simulink model "UserVehicle_RTW"  (Simulink 10.3)
settings: Solver=ode1  StartTime=0.0  StopTime=inf  FixedStep=0.001  RelTol=1e-3
PreLoadFcn:
  | vehicle = 'Car'; if ~length(which('cmcmd')), cmenv; end
  | UserVehicle_RTW_bus
  | UserVehicle_RTW_params
InitFcn:
  | vehicle = 'Car'; if ~length(which('cmcmd')), cmenv; end
  | UserVehicle_RTW_bus
undefined symbols (not defined in the file or in its folder): Car_Bdy1_mass, Car_Steering_i, Car_WhlBaseF, Car_WhlBaseR
libraries: CarMaker4SL x77
(part 1 of 3)
Description:
  | CarMaker Plug-in Model Target
settings Model: Creator=IPG  LastModifiedBy=IPG  MultithreadedSim=on
settings DataIOCC: LimitDataPoints=on
settings DebuggingCC: SFExecutionAtInitializationDiag=warning
settings HardwareCC: TargetHWDeviceType=32-bit Generic  ProdEqTarget=off
settings RTWCC: Description=CarMaker Plug-in Model Target  SystemTargetFile=CarMaker.tlc  TemplateMakefile=CarMaker_unix-win64.tmf
settings CodeAppCC: MaxIdLength=127
settings STFCustomTargetCC: ModelReferenceCompliant=off  CodeInterfacePackaging=Reusable function  CPPClassGenCompliant=on  GRTInterface=off  GenerateAllocFcn=on  SystemTargetFile=CarMaker.tlc
settings GRTTargetCC: ModelReferenceCompliant=off  ParMdlRefBuildCompliant=off  CompOptLevelCompliant=off  ConcurrentExecutionCompliant=off  MatFileLogging=off  CodeInterfacePackaging=Reusable function  GRTInterface=off  GenerateAllocFcn=on  UseToolchainInfoCompliant=off
settings CustomProperty: DataType=string
settings EnumStrPairs: String=Car

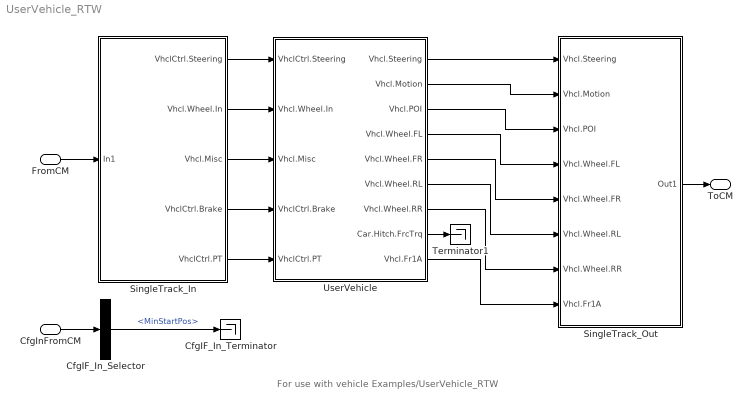
== system UserVehicle_RTW ==
  note: For use with vehicle Examples/UserVehicle_RTW
  FromCM : Inport  OutDataTypeStr=Bus: cmVehicle_CarIn
  CfgInFromCM : Inport  Port=2  OutDataTypeStr=Bus: cmVehicle_CarCfgIn
  CfgIF_In_Selector : BusSelector  OutputSignals=MinStartPos
  CfgIF_In_Terminator : Terminator
  SingleTrack_In : Subsystem
  SingleTrack_Out : Subsystem
  Terminator1 : Terminator
  UserVehicle : Subsystem
  ToCM : Outport  OutDataTypeStr=Bus: cmVehicle_CarOut  VectorParamsAs1DForOutWhenUnconnected=off
  wires:
  FromCM/1 -> SingleTrack_In/1(In1)
  SingleTrack_Out/1(Out1) -> ToCM/1
  CfgInFromCM/1 -> CfgIF_In_Selector/1
  CfgIF_In_Selector/1 -> CfgIF_In_Terminator/1  "<MinStartPos>"
  SingleTrack_In/1(VhclCtrl.Steering) -> UserVehicle/1(VhclCtrl.Steering)
  SingleTrack_In/2(Vhcl.Wheel.In) -> UserVehicle/2(Vhcl.Wheel.In)
  SingleTrack_In/3(Vhcl.Misc) -> UserVehicle/3(Vhcl.Misc)
  SingleTrack_In/4(VhclCtrl.Brake) -> UserVehicle/4(VhclCtrl.Brake)
  SingleTrack_In/5(VhclCtrl.PT) -> UserVehicle/5(VhclCtrl.PT)
  UserVehicle/1(Vhcl.Steering) -> SingleTrack_Out/1(Vhcl.Steering)
  UserVehicle/2(Vhcl.Motion) -> SingleTrack_Out/2(Vhcl.Motion)
  UserVehicle/3(Vhcl.POI) -> SingleTrack_Out/3(Vhcl.POI)
  UserVehicle/4(Vhcl.Wheel.FL) -> SingleTrack_Out/4(Vhcl.Wheel.FL)
  UserVehicle/5(Vhcl.Wheel.FR) -> SingleTrack_Out/5(Vhcl.Wheel.FR)
  UserVehicle/6(Vhcl.Wheel.RL) -> SingleTrack_Out/6(Vhcl.Wheel.RL)
  UserVehicle/7(Vhcl.Wheel.RR) -> SingleTrack_Out/7(Vhcl.Wheel.RR)
  UserVehicle/9(Vhcl.Fr1A) -> SingleTrack_Out/8(Vhcl.Fr1A)
  UserVehicle/8(Car.Hitch.FrcTrq) -> Terminator1/1

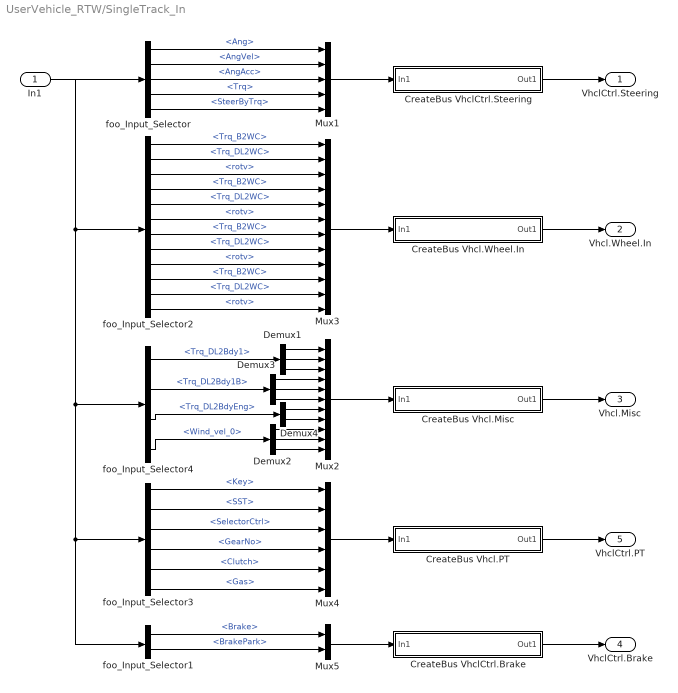
== system UserVehicle_RTW/SingleTrack_In ==
  In1 : Inport
  CreateBus Vhcl.Misc : Subsystem
  CreateBus Vhcl.PT : Subsystem
  CreateBus Vhcl.Wheel.In : Subsystem
  CreateBus VhclCtrl.Brake : Subsystem
  CreateBus VhclCtrl.Steering : Subsystem
  Demux1 : Demux  Outputs=3
      settings: DisplayOption=none
  Demux2 : Demux  Outputs=3
      settings: DisplayOption=none
  Demux3 : Demux  Outputs=3
      settings: DisplayOption=none
  Demux4 : Demux  Outputs=2
      settings: DisplayOption=none
  Mux1 : Mux  Inputs=5
  Mux2 : Mux  Inputs=11
  Mux3 : Mux  Inputs=12
  Mux4 : Mux  Inputs=6
  Mux5 : Mux  Inputs=2
  foo_Input_Selector : BusSelector  OutputSignals=VhclCtrl.Steering.Ang,VhclCtrl.Steering.AngVel,VhclCtrl.Steering.AngAcc,VhclCtrl.Steering.Trq,VhclCtrl.Steering.SteerByTrq
  foo_Input_Selector1 : BusSelector  OutputSignals=VhclCtrl.Brake,VhclCtrl.BrakePark
  foo_Input_Selector2 : BusSelector  OutputSignals=Vhcl.Wheel.FL.Trq_B2WC,Vhcl.Wheel.FL.Trq_DL2WC,Vhcl.Wheel.FL.rotv,Vhcl.Wheel.FR.Trq_B2WC,Vhcl.Wheel.FR.Trq_DL2WC,Vhcl.Wheel.FR.rotv,Vhcl.Wheel.RL.Trq_B2WC,Vhcl.Wheel.RL.Trq_DL2WC,Vhcl.Wheel.RL.rotv,Vhcl.Wheel.RR.Trq_B2WC,Vhcl.Wheel.RR.Trq_DL2WC,Vhcl.Wheel.RR.rotv
  foo_Input_Selector3 : BusSelector  OutputSignals=VhclCtrl.Key,VhclCtrl.SST,VhclCtrl.SelectorCtrl,VhclCtrl.GearNo,VhclCtrl.Clutch,VhclCtrl.Gas
  foo_Input_Selector4 : BusSelector  OutputSignals=Vhcl.Trq_DL2Bdy1,Vhcl.Trq_DL2Bdy1B,Vhcl.Trq_DL2BdyEng,Vhcl.Wind_vel_0
  VhclCtrl.Steering : Outport  VectorParamsAs1DForOutWhenUnconnected=off
  Vhcl.Wheel.In : Outport  Port=2  VectorParamsAs1DForOutWhenUnconnected=off
  Vhcl.Misc : Outport  Port=3  VectorParamsAs1DForOutWhenUnconnected=off
  VhclCtrl.Brake : Outport  Port=4  VectorParamsAs1DForOutWhenUnconnected=off
  VhclCtrl.PT : Outport  Port=5  VectorParamsAs1DForOutWhenUnconnected=off
  wires:
  foo_Input_Selector4/3 -> Demux4/1  "<Trq_DL2BdyEng>"
  Demux4/2 -> Mux2/8
  Demux4/1 -> Mux2/7
  foo_Input_Selector4/2 -> Demux3/1  "<Trq_DL2Bdy1B>"
  foo_Input_Selector4/1 -> Demux1/1  "<Trq_DL2Bdy1>"
  Demux3/3 -> Mux2/6
  Demux3/2 -> Mux2/5
  Demux3/1 -> Mux2/4
  Demux1/3 -> Mux2/3
  Demux1/2 -> Mux2/2
  Demux1/1 -> Mux2/1
  Demux2/3 -> Mux2/11
  Demux2/2 -> Mux2/10
  Demux2/1 -> Mux2/9
  foo_Input_Selector4/4 -> Demux2/1  "<Wind_vel_0>"
  foo_Input_Selector/5 -> Mux1/5  "<SteerByTrq>"
  In1/1 -> foo_Input_Selector4/1, foo_Input_Selector1/1, foo_Input_Selector3/1, foo_Input_Selector/1, foo_Input_Selector2/1
  foo_Input_Selector/1 -> Mux1/1  "<Ang>"
  foo_Input_Selector/2 -> Mux1/2  "<AngVel>"
  foo_Input_Selector/3 -> Mux1/3  "<AngAcc>"
  foo_Input_Selector/4 -> Mux1/4  "<Trq>"
  foo_Input_Selector2/1 -> Mux3/1  "<Trq_B2WC>"
  foo_Input_Selector2/2 -> Mux3/2  "<Trq_DL2WC>"
  foo_Input_Selector2/3 -> Mux3/3  "<rotv>"
  foo_Input_Selector2/4 -> Mux3/4  "<Trq_B2WC>"
  foo_Input_Selector2/5 -> Mux3/5  "<Trq_DL2WC>"
  foo_Input_Selector2/6 -> Mux3/6  "<rotv>"
  foo_Input_Selector2/7 -> Mux3/7  "<Trq_B2WC>"
  foo_Input_Selector2/8 -> Mux3/8  "<Trq_DL2WC>"
  foo_Input_Selector2/9 -> Mux3/9  "<rotv>"
  foo_Input_Selector2/10 -> Mux3/10  "<Trq_B2WC>"
  foo_Input_Selector2/11 -> Mux3/11  "<Trq_DL2WC>"
  foo_Input_Selector2/12 -> Mux3/12  "<rotv>"
  foo_Input_Selector1/1 -> Mux5/1  "<Brake>"
  Mux1/1 -> CreateBus VhclCtrl.Steering/1(In1)
  CreateBus VhclCtrl.Steering/1(Out1) -> VhclCtrl.Steering/1
  Mux3/1 -> CreateBus Vhcl.Wheel.In/1(In1)
  CreateBus Vhcl.Wheel.In/1(Out1) -> Vhcl.Wheel.In/1
  Mux2/1 -> CreateBus Vhcl.Misc/1(In1)
  CreateBus Vhcl.Misc/1(Out1) -> Vhcl.Misc/1
  Mux4/1 -> CreateBus Vhcl.PT/1(In1)
  CreateBus Vhcl.PT/1(Out1) -> VhclCtrl.PT/1
  Mux5/1 -> CreateBus VhclCtrl.Brake/1(In1)
  CreateBus VhclCtrl.Brake/1(Out1) -> VhclCtrl.Brake/1
  foo_Input_Selector1/2 -> Mux5/2  "<BrakePark>"
  foo_Input_Selector3/1 -> Mux4/1  "<Key>"
  foo_Input_Selector3/2 -> Mux4/2  "<SST>"
  foo_Input_Selector3/3 -> Mux4/3  "<SelectorCtrl>"
  foo_Input_Selector3/4 -> Mux4/4  "<GearNo>"
  foo_Input_Selector3/5 -> Mux4/5  "<Clutch>"
  foo_Input_Selector3/6 -> Mux4/6  "<Gas>"

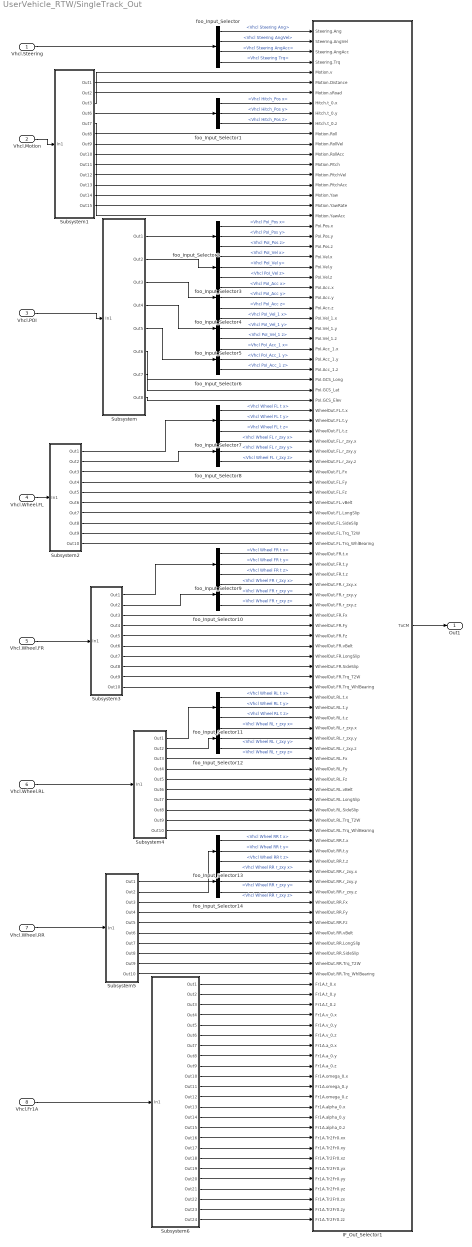
== system UserVehicle_RTW/SingleTrack_Out ==
  Vhcl.Steering : Inport
  Vhcl.Motion : Inport  Port=2
  Vhcl.POI : Inport  Port=3
  Vhcl.Wheel.FL : Inport  Port=4
  Vhcl.Wheel.FR : Inport  Port=5
  Vhcl.Wheel.RL : Inport  Port=6
  Vhcl.Wheel.RR : Inport  Port=7
  Vhcl.Fr1A : Inport  Port=8
  IF_Out_Selector1 : Subsystem  mask(Signal Selection){}
      mask help: Signal Selection Block
      settings: OpenFcn=cmSignalSelect('SignalSelection_CB',gcb)
  Subsystem : Subsystem
  Subsystem1 : Subsystem
  Subsystem2 : Subsystem
  Subsystem3 : Subsystem
  Subsystem4 : Subsystem
  Subsystem5 : Subsystem
  Subsystem6 : Subsystem
  foo_Input_Selector : BusSelector  OutputSignals=Vhcl Steering Ang,Vhcl Steering AngVel,Vhcl Steering AngAcc,Vhcl Steering Trq
  foo_Input_Selector1 : BusSelector  OutputSignals=Vhcl Hitch_Pos x,Vhcl Hitch_Pos y,Vhcl Hitch_Pos z
  foo_Input_Selector10 : BusSelector  OutputSignals=Vhcl Wheel FR r_zxy x,Vhcl Wheel FR r_zxy y,Vhcl Wheel FR r_zxy z
  foo_Input_Selector11 : BusSelector  OutputSignals=Vhcl Wheel RL t x,Vhcl Wheel RL t y,Vhcl Wheel RL t z
  foo_Input_Selector12 : BusSelector  OutputSignals=Vhcl Wheel RL r_zxy x,Vhcl Wheel RL r_zxy y,Vhcl Wheel RL r_zxy z
  foo_Input_Selector13 : BusSelector  OutputSignals=Vhcl Wheel RR t x,Vhcl Wheel RR t y,Vhcl Wheel RR t z
  foo_Input_Selector14 : BusSelector  OutputSignals=Vhcl Wheel RR r_zxy x,Vhcl Wheel RR r_zxy y,Vhcl Wheel RR r_zxy z
  foo_Input_Selector2 : BusSelector  OutputSignals=Vhcl PoI_Pos x,Vhcl PoI_Pos y,Vhcl PoI_Pos z
  foo_Input_Selector3 : BusSelector  OutputSignals=Vhcl PoI_Vel x,Vhcl PoI_Vel y,Vhcl PoI_Vel z
  foo_Input_Selector4 : BusSelector  OutputSignals=Vhcl PoI_Acc x,Vhcl PoI_Acc y,Vhcl PoI_Acc z
  foo_Input_Selector5 : BusSelector  OutputSignals=Vhcl PoI_Vel_1 x,Vhcl PoI_Vel_1 y,Vhcl PoI_Vel_1 z
  foo_Input_Selector6 : BusSelector  OutputSignals=Vhcl PoI_Acc_1 x,Vhcl PoI_Acc_1 y,Vhcl PoI_Acc_1 z
  foo_Input_Selector7 : BusSelector  OutputSignals=Vhcl Wheel FL t x,Vhcl Wheel FL t y,Vhcl Wheel FL t z
  foo_Input_Selector8 : BusSelector  OutputSignals=Vhcl Wheel FL r_zxy x,Vhcl Wheel FL r_zxy y,Vhcl Wheel FL r_zxy z
  foo_Input_Selector9 : BusSelector  OutputSignals=Vhcl Wheel FR t x,Vhcl Wheel FR t y,Vhcl Wheel FR t z
  Out1 : Outport  VectorParamsAs1DForOutWhenUnconnected=off
  wires:
  Subsystem5/2(Out2) -> foo_Input_Selector14/1
  Subsystem5/1(Out1) -> foo_Input_Selector13/1
  Subsystem4/2(Out2) -> foo_Input_Selector12/1
  Subsystem4/1(Out1) -> foo_Input_Selector11/1
  Subsystem3/2(Out2) -> foo_Input_Selector10/1
  Subsystem3/1(Out1) -> foo_Input_Selector9/1
  Subsystem2/2(Out2) -> foo_Input_Selector8/1
  Subsystem2/1(Out1) -> foo_Input_Selector7/1
  Subsystem/5(Out5) -> foo_Input_Selector6/1
  Subsystem/4(Out4) -> foo_Input_Selector5/1
  Subsystem/3(Out3) -> foo_Input_Selector4/1
  Subsystem/2(Out2) -> foo_Input_Selector3/1
  Subsystem/1(Out1) -> foo_Input_Selector2/1
  Vhcl.Steering/1 -> foo_Input_Selector/1
  Vhcl.Motion/1 -> Subsystem1/1(In1)
  Vhcl.POI/1 -> Subsystem/1(In1)
  Vhcl.Wheel.FL/1 -> Subsystem2/1(In1)
  Vhcl.Wheel.FR/1 -> Subsystem3/1(In1)
  Vhcl.Wheel.RL/1 -> Subsystem4/1(In1)
  Vhcl.Wheel.RR/1 -> Subsystem5/1(In1)
  Vhcl.Fr1A/1 -> Subsystem6/1(In1)
  Subsystem1/4(Out6) -> foo_Input_Selector1/1
  foo_Input_Selector/1 -> IF_Out_Selector1/1(Steering.Ang)  "<Vhcl Steering Ang>"
  foo_Input_Selector/2 -> IF_Out_Selector1/2(Steering.AngVel)  "<Vhcl Steering AngVel>"
  foo_Input_Selector/3 -> IF_Out_Selector1/3(Steering.AngAcc)  "<Vhcl Steering AngAcc>"
  foo_Input_Selector/4 -> IF_Out_Selector1/4(Steering.Trq)  "<Vhcl Steering Trq>"
  Subsystem1/1(Out1) -> IF_Out_Selector1/5(Motion.v)
  Subsystem1/2(Out2) -> IF_Out_Selector1/6(Motion.Distance)
  Subsystem1/3(Out3) -> IF_Out_Selector1/7(Motion.sRoad)
  foo_Input_Selector1/1 -> IF_Out_Selector1/8(Hitch.t_0.x)  "<Vhcl Hitch_Pos x>"
  foo_Input_Selector1/2 -> IF_Out_Selector1/9(Hitch.t_0.y)  "<Vhcl Hitch_Pos y>"
  foo_Input_Selector1/3 -> IF_Out_Selector1/10(Hitch.t_0.z)  "<Vhcl Hitch_Pos z>"
  Subsystem1/5(Out7) -> IF_Out_Selector1/11(Motion.Roll)
  Subsystem1/6(Out8) -> IF_Out_Selector1/12(Motion.RollVel)
  Subsystem1/7(Out9) -> IF_Out_Selector1/13(Motion.RollAcc)
  Subsystem1/8(Out10) -> IF_Out_Selector1/14(Motion.Pitch)
  Subsystem1/9(Out11) -> IF_Out_Selector1/15(Motion.PitchVel)
  Subsystem1/10(Out12) -> IF_Out_Selector1/16(Motion.PitchAcc)
  Subsystem1/11(Out13) -> IF_Out_Selector1/17(Motion.Yaw)
  Subsystem1/12(Out14) -> IF_Out_Selector1/18(Motion.YawRate)
  Subsystem1/13(Out15) -> IF_Out_Selector1/19(Motion.YawAcc)
  foo_Input_Selector2/1 -> IF_Out_Selector1/20(PoI.Pos.x)  "<Vhcl PoI_Pos x>"
  foo_Input_Selector2/2 -> IF_Out_Selector1/21(PoI.Pos.y)  "<Vhcl PoI_Pos y>"
  foo_Input_Selector2/3 -> IF_Out_Selector1/22(PoI.Pos.z)  "<Vhcl PoI_Pos z>"
  foo_Input_Selector3/1 -> IF_Out_Selector1/23(PoI.Vel.x)  "<Vhcl PoI_Vel x>"
  foo_Input_Selector3/2 -> IF_Out_Selector1/24(PoI.Vel.y)  "<Vhcl PoI_Vel y>"
  foo_Input_Selector3/3 -> IF_Out_Selector1/25(PoI.Vel.z)  "<Vhcl PoI_Vel z>"
  foo_Input_Selector4/1 -> IF_Out_Selector1/26(PoI.Acc.x)  "<Vhcl PoI_Acc x>"
  foo_Input_Selector4/2 -> IF_Out_Selector1/27(PoI.Acc.y)  "<Vhcl PoI_Acc y>"
  foo_Input_Selector4/3 -> IF_Out_Selector1/28(PoI.Acc.z)  "<Vhcl PoI_Acc z>"
  foo_Input_Selector5/1 -> IF_Out_Selector1/29(PoI.Vel_1.x)  "<Vhcl PoI_Vel_1 x>"
  foo_Input_Selector5/2 -> IF_Out_Selector1/30(PoI.Vel_1.y)  "<Vhcl PoI_Vel_1 y>"
  foo_Input_Selector5/3 -> IF_Out_Selector1/31(PoI.Vel_1.z)  "<Vhcl PoI_Vel_1 z>"
  foo_Input_Selector6/1 -> IF_Out_Selector1/32(PoI.Acc_1.x)  "<Vhcl PoI_Acc_1 x>"
  foo_Input_Selector6/2 -> IF_Out_Selector1/33(PoI.Acc_1.y)  "<Vhcl PoI_Acc_1 y>"
  foo_Input_Selector6/3 -> IF_Out_Selector1/34(PoI.Acc_1.z)  "<Vhcl PoI_Acc_1 z>"
  Subsystem/6(Out6) -> IF_Out_Selector1/35(PoI.GCS_Long)
  Subsystem/7(Out7) -> IF_Out_Selector1/36(PoI.GCS_Lat)
  Subsystem/8(Out8) -> IF_Out_Selector1/37(PoI.GCS_Elev)
  foo_Input_Selector7/1 -> IF_Out_Selector1/38(WheelOut.FL.t.x)  "<Vhcl Wheel FL t x>"
  foo_Input_Selector7/2 -> IF_Out_Selector1/39(WheelOut.FL.t.y)  "<Vhcl Wheel FL t y>"
  foo_Input_Selector7/3 -> IF_Out_Selector1/40(WheelOut.FL.t.z)  "<Vhcl Wheel FL t z>"
  foo_Input_Selector8/1 -> IF_Out_Selector1/41(WheelOut.FL.r_zxy.x)  "<Vhcl Wheel FL r_zxy x>"
  foo_Input_Selector8/2 -> IF_Out_Selector1/42(WheelOut.FL.r_zxy.y)  "<Vhcl Wheel FL r_zxy y>"
  foo_Input_Selector8/3 -> IF_Out_Selector1/43(WheelOut.FL.r_zxy.z)  "<Vhcl Wheel FL r_zxy z>"
  Subsystem2/3(Out3) -> IF_Out_Selector1/44(WheelOut.FL.Fx)
  Subsystem2/4(Out4) -> IF_Out_Selector1/45(WheelOut.FL.Fy)
  Subsystem2/5(Out5) -> IF_Out_Selector1/46(WheelOut.FL.Fz)
  Subsystem2/6(Out6) -> IF_Out_Selector1/47(WheelOut.FL.vBelt)
  Subsystem2/7(Out7) -> IF_Out_Selector1/48(WheelOut.FL.LongSlip)
  Subsystem2/8(Out8) -> IF_Out_Selector1/49(WheelOut.FL.SideSlip)
  Subsystem2/9(Out9) -> IF_Out_Selector1/50(WheelOut.FL.Trq_T2W)
  Subsystem2/10(Out10) -> IF_Out_Selector1/51(WheelOut.FL.Trq_WhlBearing)
  foo_Input_Selector9/1 -> IF_Out_Selector1/52(WheelOut.FR.t.x)  "<Vhcl Wheel FR t x>"
  foo_Input_Selector9/2 -> IF_Out_Selector1/53(WheelOut.FR.t.y)  "<Vhcl Wheel FR t y>"
  foo_Input_Selector9/3 -> IF_Out_Selector1/54(WheelOut.FR.t.z)  "<Vhcl Wheel FR t z>"
  foo_Input_Selector10/1 -> IF_Out_Selector1/55(WheelOut.FR.r_zxy.x)  "<Vhcl Wheel FR r_zxy x>"
  foo_Input_Selector10/2 -> IF_Out_Selector1/56(WheelOut.FR.r_zxy.y)  "<Vhcl Wheel FR r_zxy y>"
  foo_Input_Selector10/3 -> IF_Out_Selector1/57(WheelOut.FR.r_zxy.z)  "<Vhcl Wheel FR r_zxy z>"
  Subsystem3/3(Out3) -> IF_Out_Selector1/58(WheelOut.FR.Fx)
  Subsystem3/4(Out4) -> IF_Out_Selector1/59(WheelOut.FR.Fy)
  Subsystem3/5(Out5) -> IF_Out_Selector1/60(WheelOut.FR.Fz)
  Subsystem3/6(Out6) -> IF_Out_Selector1/61(WheelOut.FR.vBelt)
  Subsystem3/7(Out7) -> IF_Out_Selector1/62(WheelOut.FR.LongSlip)
  Subsystem3/8(Out8) -> IF_Out_Selector1/63(WheelOut.FR.SideSlip)
  Subsystem3/9(Out9) -> IF_Out_Selector1/64(WheelOut.FR.Trq_T2W)
  Subsystem3/10(Out10) -> IF_Out_Selector1/65(WheelOut.FR.Trq_WhlBearing)
  foo_Input_Selector11/1 -> IF_Out_Selector1/66(WheelOut.RL.t.x)  "<Vhcl Wheel RL t x>"
  foo_Input_Selector11/2 -> IF_Out_Selector1/67(WheelOut.RL.t.y)  "<Vhcl Wheel RL t y>"
  foo_Input_Selector11/3 -> IF_Out_Selector1/68(WheelOut.RL.t.z)  "<Vhcl Wheel RL t z>"
  foo_Input_Selector12/1 -> IF_Out_Selector1/69(WheelOut.RL.r_zxy.x)  "<Vhcl Wheel RL r_zxy x>"
  foo_Input_Selector12/2 -> IF_Out_Selector1/70(WheelOut.RL.r_zxy.y)  "<Vhcl Wheel RL r_zxy y>"
  foo_Input_Selector12/3 -> IF_Out_Selector1/71(WheelOut.RL.r_zxy.z)  "<Vhcl Wheel RL r_zxy z>"
  Subsystem4/3(Out3) -> IF_Out_Selector1/72(WheelOut.RL.Fx)
  Subsystem4/4(Out4) -> IF_Out_Selector1/73(WheelOut.RL.Fy)
  Subsystem4/5(Out5) -> IF_Out_Selector1/74(WheelOut.RL.Fz)
  Subsystem4/6(Out6) -> IF_Out_Selector1/75(WheelOut.RL.vBelt)
  Subsystem4/7(Out7) -> IF_Out_Selector1/76(WheelOut.RL.LongSlip)
  Subsystem4/8(Out8) -> IF_Out_Selector1/77(WheelOut.RL.SideSlip)
  Subsystem4/9(Out9) -> IF_Out_Selector1/78(WheelOut.RL.Trq_T2W)
  Subsystem4/10(Out10) -> IF_Out_Selector1/79(WheelOut.RL.Trq_WhlBearing)
  foo_Input_Selector13/1 -> IF_Out_Selector1/80(WheelOut.RR.t.x)  "<Vhcl Wheel RR t x>"
  foo_Input_Selector13/2 -> IF_Out_Selector1/81(WheelOut.RR.t.y)  "<Vhcl Wheel RR t y>"
  foo_Input_Selector13/3 -> IF_Out_Selector1/82(WheelOut.RR.t.z)  "<Vhcl Wheel RR t z>"
  foo_Input_Selector14/1 -> IF_Out_Selector1/83(WheelOut.RR.r_zxy.x)  "<Vhcl Wheel RR r_zxy x>"
  foo_Input_Selector14/2 -> IF_Out_Selector1/84(WheelOut.RR.r_zxy.y)  "<Vhcl Wheel RR r_zxy y>"
  foo_Input_Selector14/3 -> IF_Out_Selector1/85(WheelOut.RR.r_zxy.z)  "<Vhcl Wheel RR r_zxy z>"
  Subsystem5/3(Out3) -> IF_Out_Selector1/86(WheelOut.RR.Fx)
  Subsystem5/4(Out4) -> IF_Out_Selector1/87(WheelOut.RR.Fy)
  Subsystem5/5(Out5) -> IF_Out_Selector1/88(WheelOut.RR.Fz)
  Subsystem5/6(Out6) -> IF_Out_Selector1/89(WheelOut.RR.vBelt)
  Subsystem5/7(Out7) -> IF_Out_Selector1/90(WheelOut.RR.LongSlip)
  Subsystem5/8(Out8) -> IF_Out_Selector1/91(WheelOut.RR.SideSlip)
  Subsystem5/9(Out9) -> IF_Out_Selector1/92(WheelOut.RR.Trq_T2W)
  Subsystem5/10(Out10) -> IF_Out_Selector1/93(WheelOut.RR.Trq_WhlBearing)
  Subsystem6/1(Out1) -> IF_Out_Selector1/94(Fr1A.t_0.x)
  Subsystem6/2(Out2) -> IF_Out_Selector1/95(Fr1A.t_0.y)
  Subsystem6/3(Out3) -> IF_Out_Selector1/96(Fr1A.t_0.z)
  Subsystem6/4(Out4) -> IF_Out_Selector1/97(Fr1A.v_0.x)
  Subsystem6/5(Out5) -> IF_Out_Selector1/98(Fr1A.v_0.y)
  Subsystem6/6(Out6) -> IF_Out_Selector1/99(Fr1A.v_0.z)
  Subsystem6/7(Out7) -> IF_Out_Selector1/100(Fr1A.a_0.x)
  Subsystem6/8(Out8) -> IF_Out_Selector1/101(Fr1A.a_0.y)
  Subsystem6/9(Out9) -> IF_Out_Selector1/102(Fr1A.a_0.z)
  Subsystem6/10(Out10) -> IF_Out_Selector1/103(Fr1A.omega_0.x)
  Subsystem6/11(Out11) -> IF_Out_Selector1/104(Fr1A.omega_0.y)
  Subsystem6/12(Out12) -> IF_Out_Selector1/105(Fr1A.omega_0.z)
  Subsystem6/13(Out13) -> IF_Out_Selector1/106(Fr1A.alpha_0.x)
  Subsystem6/14(Out14) -> IF_Out_Selector1/107(Fr1A.alpha_0.y)
  Subsystem6/15(Out15) -> IF_Out_Selector1/108(Fr1A.alpha_0.z)
  Subsystem6/16(Out16) -> IF_Out_Selector1/109(Fr1A.Tr2Fr0.xx)
  Subsystem6/17(Out17) -> IF_Out_Selector1/110(Fr1A.Tr2Fr0.xy)
  Subsystem6/18(Out18) -> IF_Out_Selector1/111(Fr1A.Tr2Fr0.xz)
  Subsystem6/19(Out19) -> IF_Out_Selector1/112(Fr1A.Tr2Fr0.yx)
  Subsystem6/20(Out20) -> IF_Out_Selector1/113(Fr1A.Tr2Fr0.yy)
  Subsystem6/21(Out21) -> IF_Out_Selector1/114(Fr1A.Tr2Fr0.yz)
  Subsystem6/22(Out22) -> IF_Out_Selector1/115(Fr1A.Tr2Fr0.zx)
  Subsystem6/23(Out23) -> IF_Out_Selector1/116(Fr1A.Tr2Fr0.zy)
  Subsystem6/24(Out24) -> IF_Out_Selector1/117(Fr1A.Tr2Fr0.zz)
  IF_Out_Selector1/1(ToCM) -> Out1/1

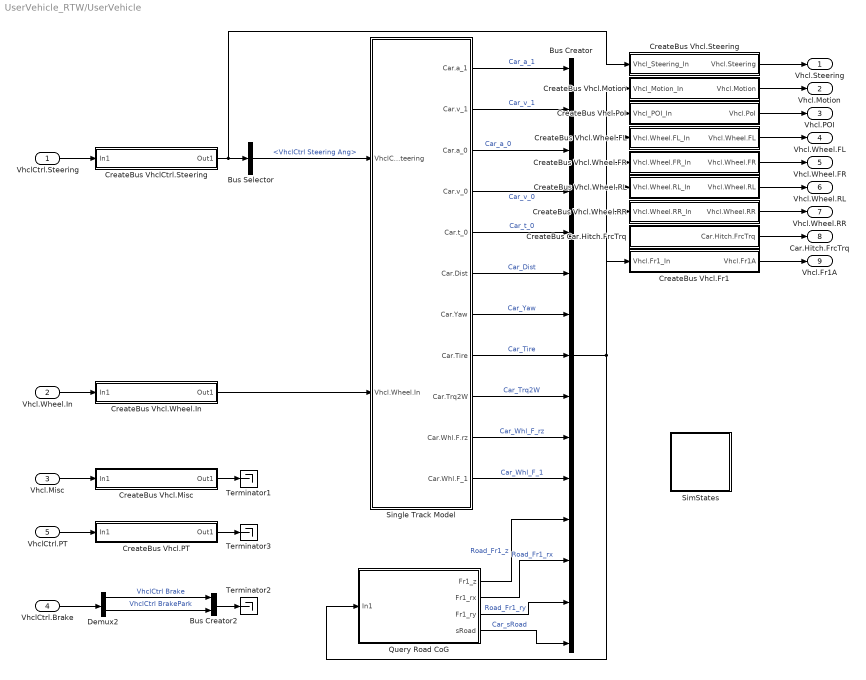
== system UserVehicle_RTW/UserVehicle ==
  VhclCtrl.Steering : Inport  OutDataTypeStr=double  BusOutputAsStruct=on
  Vhcl.Wheel.In : Inport  Port=2
  Vhcl.Misc : Inport  Port=3
  VhclCtrl.Brake : Inport  Port=4
  VhclCtrl.PT : Inport  Port=5
  Bus Creator : BusCreator  Inputs=15
  Bus Creator2 : BusCreator  Inputs=2
  Bus Selector : BusSelector  OutputSignals=VhclCtrl Steering Ang
  CreateBus Car.Hitch.FrcTrq : Subsystem
  CreateBus Vhcl.Fr1 : Subsystem
  CreateBus Vhcl.Misc : Subsystem
  CreateBus Vhcl.Motion : Subsystem
  CreateBus Vhcl.PT : Subsystem
  CreateBus Vhcl.PoI : Subsystem
  CreateBus Vhcl.Steering : Subsystem
  CreateBus Vhcl.Wheel.FL : Subsystem
  CreateBus Vhcl.Wheel.FR : Subsystem
  CreateBus Vhcl.Wheel.In : Subsystem
  CreateBus Vhcl.Wheel.RL : Subsystem
  CreateBus Vhcl.Wheel.RR : Subsystem
  CreateBus VhclCtrl.Steering : Subsystem
  Demux2 : Demux  Outputs=2
      settings: DisplayOption=none
  Query Road CoG : Subsystem
  SimStates : Subsystem
  Single Track Model : Subsystem
  Terminator1 : Terminator
  Terminator2 : Terminator
  Terminator3 : Terminator
  Vhcl.Steering : Outport  VectorParamsAs1DForOutWhenUnconnected=off
  Vhcl.Motion : Outport  Port=2  VectorParamsAs1DForOutWhenUnconnected=off
  Vhcl.POI : Outport  Port=3  VectorParamsAs1DForOutWhenUnconnected=off
  Vhcl.Wheel.FL : Outport  Port=4  VectorParamsAs1DForOutWhenUnconnected=off
  Vhcl.Wheel.FR : Outport  Port=5  VectorParamsAs1DForOutWhenUnconnected=off
  Vhcl.Wheel.RL : Outport  Port=6  VectorParamsAs1DForOutWhenUnconnected=off
  Vhcl.Wheel.RR : Outport  Port=7  VectorParamsAs1DForOutWhenUnconnected=off
  Car.Hitch.FrcTrq : Outport  Port=8  VectorParamsAs1DForOutWhenUnconnected=off
  Vhcl.Fr1A : Outport  Port=9  VectorParamsAs1DForOutWhenUnconnected=off
  wires:
  CreateBus Vhcl.Wheel.In/1(Out1) -> Single Track Model/2(Vhcl.Wheel.In)
  Single Track Model/11(Car.Whl.F_1) -> Bus Creator/11  "Car_Whl_F_1"
  Query Road CoG/4(sRoad) -> Bus Creator/15  "Car_sRoad"
  Query Road CoG/3(Fr1_ry) -> Bus Creator/14  "Road_Fr1_ry"
  Query Road CoG/2(Fr1_rx) -> Bus Creator/13  "Road_Fr1_rx"
  Query Road CoG/1(Fr1_z) -> Bus Creator/12  "Road_Fr1_z"
  Single Track Model/10(Car.Whl.F.rz) -> Bus Creator/10  "Car_Whl_F_rz"
  Bus Selector/1 -> Single Track Model/1(VhclCtrl.Steering)  "<VhclCtrl Steering Ang>"
  Single Track Model/1(Car.a_1) -> Bus Creator/1  "Car_a_1"
  Single Track Model/2(Car.v_1) -> Bus Creator/2  "Car_v_1"
  Single Track Model/3(Car.a_0) -> Bus Creator/3  "Car_a_0"
  Single Track Model/4(Car.v_0) -> Bus Creator/4  "Car_v_0"
  Single Track Model/5(Car.t_0) -> Bus Creator/5  "Car_t_0"
  Single Track Model/6(Car.Dist) -> Bus Creator/6  "Car_Dist"
  Single Track Model/7(Car.Yaw) -> Bus Creator/7  "Car_Yaw"
  Single Track Model/8(Car.Tire) -> Bus Creator/8  "Car_Tire"
  Single Track Model/9(Car.Trq2W) -> Bus Creator/9  "Car_Trq2W"
  Bus Creator/1 -> CreateBus Vhcl.Motion/1(Vhcl_Motion_In), CreateBus Vhcl.Wheel.RR/1(Vhcl.Wheel.RR_In), CreateBus Vhcl.Wheel.RL/1(Vhcl.Wheel.RL_In), CreateBus Vhcl.Wheel.FR/1(Vhcl.Wheel.FR_In), CreateBus Vhcl.Wheel.FL/1(Vhcl.Wheel.FL_In), CreateBus Vhcl.Fr1/1(Vhcl.Fr1_In), Query Road CoG/1(In1), CreateBus Vhcl.PoI/1(Vhcl_POI_In)
  CreateBus Vhcl.PT/1(Out1) -> Terminator3/1
  Bus Creator2/1 -> Terminator2/1
  CreateBus Vhcl.Misc/1(Out1) -> Terminator1/1
  VhclCtrl.Brake/1 -> Demux2/1
  Demux2/2 -> Bus Creator2/2  "VhclCtrl BrakePark"
  Demux2/1 -> Bus Creator2/1  "VhclCtrl Brake"
  CreateBus VhclCtrl.Steering/1(Out1) -> CreateBus Vhcl.Steering/1(Vhcl_Steering_In), Bus Selector/1
  VhclCtrl.Steering/1 -> CreateBus VhclCtrl.Steering/1(In1)
  Vhcl.Wheel.In/1 -> CreateBus Vhcl.Wheel.In/1(In1)
  Vhcl.Misc/1 -> CreateBus Vhcl.Misc/1(In1)
  CreateBus Vhcl.Steering/1(Vhcl.Steering) -> Vhcl.Steering/1
  CreateBus Vhcl.Wheel.RR/1(Vhcl.Wheel.RR) -> Vhcl.Wheel.RR/1
  CreateBus Car.Hitch.FrcTrq/1(Car.Hitch.FrcTrq) -> Car.Hitch.FrcTrq/1
  VhclCtrl.PT/1 -> CreateBus Vhcl.PT/1(In1)
  CreateBus Vhcl.Wheel.RL/1(Vhcl.Wheel.RL) -> Vhcl.Wheel.RL/1
  CreateBus Vhcl.Wheel.FR/1(Vhcl.Wheel.FR) -> Vhcl.Wheel.FR/1
  CreateBus Vhcl.Wheel.FL/1(Vhcl.Wheel.FL) -> Vhcl.Wheel.FL/1
  CreateBus Vhcl.PoI/1(Vhcl.PoI) -> Vhcl.POI/1
  CreateBus Vhcl.Motion/1(Vhcl.Motion) -> Vhcl.Motion/1
  CreateBus Vhcl.Fr1/1(Vhcl.Fr1A) -> Vhcl.Fr1A/1

== system UserVehicle_RTW/SingleTrack_In/CreateBus Vhcl.Misc ==
  In1 : Inport
  Bus Creator5 : BusCreator  Inputs=11
  Demux5 : Demux  Outputs=11
      settings: DisplayOption=none
  Out1 : Outport  VectorParamsAs1DForOutWhenUnconnected=off
  wires:
  Demux5/1 -> Bus Creator5/1  "Vhcl Trq_DL2Bdy1 x"
  Demux5/2 -> Bus Creator5/2  "Vhcl Trq_DL2Bdy1 y"
  Bus Creator5/1 -> Out1/1
  In1/1 -> Demux5/1
  Demux5/3 -> Bus Creator5/3  "Vhcl Trq_DL2Bdy1 z"
  Demux5/4 -> Bus Creator5/4  "Vhcl TrqDL2Bdy1B x"
  Demux5/5 -> Bus Creator5/5  "Vhcl TrqDL2Bdy1B y"
  Demux5/6 -> Bus Creator5/6  "Vhcl TrqDL2Bdy1B z"
  Demux5/7 -> Bus Creator5/7  "Vhcl DL2BdyEng x"
  Demux5/8 -> Bus Creator5/8  "Vhcl DL2BdyEng y"
  Demux5/9 -> Bus Creator5/9  "Vhcl Wind_vel_0 x"
  Demux5/10 -> Bus Creator5/10  "Vhcl Wind_vel_0 y"
  Demux5/11 -> Bus Creator5/11  "Vhcl Wind_vel_0 z"

== system UserVehicle_RTW/SingleTrack_In/CreateBus Vhcl.PT ==
  In1 : Inport
  Bus Creator3 : BusCreator  Inputs=6
  Demux3 : Demux  Outputs=6
      settings: DisplayOption=none
  Out1 : Outport  VectorParamsAs1DForOutWhenUnconnected=off
  wires:
  Demux3/6 -> Bus Creator3/6  "VhclCtrl Gas"
  Demux3/5 -> Bus Creator3/5  "VhclCtrl Clutch"
  Demux3/1 -> Bus Creator3/1  "VhclCtrl Key"
  Demux3/2 -> Bus Creator3/2  "VhclCtrl SST"
  Demux3/3 -> Bus Creator3/3  "VhclCtrl SelectorCtrl"
  Demux3/4 -> Bus Creator3/4  "VhclCtrl GearNo"
  Bus Creator3/1 -> Out1/1
  In1/1 -> Demux3/1

== system UserVehicle_RTW/SingleTrack_In/CreateBus Vhcl.Wheel.In ==
  In1 : Inport
  Bus Creator1 : BusCreator  Inputs=12
  Demux1 : Demux  Outputs=12
      settings: DisplayOption=none
  Out1 : Outport  VectorParamsAs1DForOutWhenUnconnected=off
  wires:
  Demux1/1 -> Bus Creator1/1  "Vhcl Wheel FL Trq_B2WC"
  Demux1/2 -> Bus Creator1/2  "Vhcl Wheel FL Trq_DL2WC"
  Bus Creator1/1 -> Out1/1
  In1/1 -> Demux1/1
  Demux1/3 -> Bus Creator1/3  "Vhcl Wheel FL rotv"
  Demux1/4 -> Bus Creator1/4  "Vhcl Wheel FR Trq_B2WC"
  Demux1/5 -> Bus Creator1/5  "Vhcl Wheel FR Trq_DL2WC"
  Demux1/6 -> Bus Creator1/6  "Vhcl Wheel FR rotv"
  Demux1/7 -> Bus Creator1/7  "Vhcl Wheel RL Trq_B2WC"
  Demux1/8 -> Bus Creator1/8  "Vhcl Wheel RL Trq_DL2WC"
  Demux1/9 -> Bus Creator1/9  "Vhcl Wheel RL rotv"
  Demux1/10 -> Bus Creator1/10  "Vhcl Wheel RR Trq_B2WC"
  Demux1/11 -> Bus Creator1/11  "Vhcl Wheel RR Trq_DL2WC"
  Demux1/12 -> Bus Creator1/12  "Vhcl Wheel RR rotv"

== system UserVehicle_RTW/SingleTrack_In/CreateBus VhclCtrl.Brake ==
  In1 : Inport
  Bus Creator2 : BusCreator  Inputs=2
  Demux2 : Demux  Outputs=2
      settings: DisplayOption=none
  Out1 : Outport  VectorParamsAs1DForOutWhenUnconnected=off
  wires:
  In1/1 -> Demux2/1
  Bus Creator2/1 -> Out1/1
  Demux2/1 -> Bus Creator2/1  "VhclCtrl Brake"
  Demux2/2 -> Bus Creator2/2  "VhclCtrl BrakePark"

== system UserVehicle_RTW/SingleTrack_In/CreateBus VhclCtrl.Steering ==
  In1 : Inport
  Bus Creator : BusCreator  Inputs=5
  Demux : Demux  Outputs=5
      settings: DisplayOption=none
  Out1 : Outport  VectorParamsAs1DForOutWhenUnconnected=off
  wires:
  Demux/4 -> Bus Creator/4  "VhclCtrl Steering Trq"
  Demux/2 -> Bus Creator/2  "VhclCtrl Steering AngVel"
  Demux/3 -> Bus Creator/3  "VhclCtrl Steering AngAcc"
  Demux/5 -> Bus Creator/5  "VhclCtrl Steering ByTrq"
  Demux/1 -> Bus Creator/1  "VhclCtrl Steering Ang"
  Bus Creator/1 -> Out1/1
  In1/1 -> Demux/1

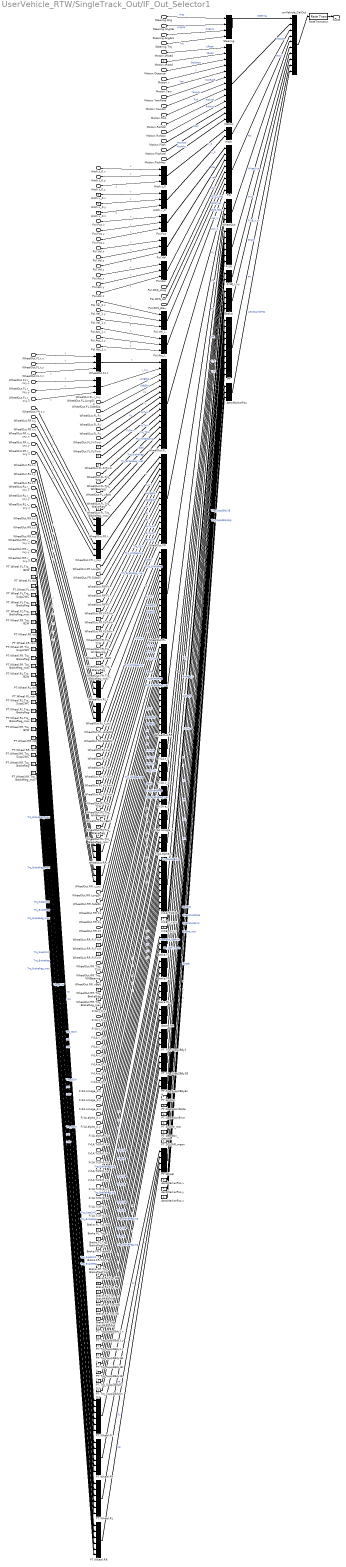
== system UserVehicle_RTW/SingleTrack_Out/IF_Out_Selector1 ==
  Steering.Ang : Inport
  Steering.AngVel : Inport  Port=2
  Steering.AngAcc : Inport  Port=3
  Steering.Trq : Inport  Port=4
  Motion.v : Inport  Port=5
  Motion.Distance : Inport  Port=6
  Motion.sRoad : Inport  Port=7
  Hitch.t_0.x : Inport  Port=8
  Hitch.t_0.y : Inport  Port=9
  Hitch.t_0.z : Inport  Port=10
  Motion.Roll : Inport  Port=11
  Motion.RollVel : Inport  Port=12
  Motion.RollAcc : Inport  Port=13
  Motion.Pitch : Inport  Port=14
  Motion.PitchVel : Inport  Port=15
  Motion.PitchAcc : Inport  Port=16
  Motion.Yaw : Inport  Port=17
  Motion.YawRate : Inport  Port=18
  Motion.YawAcc : Inport  Port=19
  PoI.Pos.x : Inport  Port=20
  PoI.Pos.y : Inport  Port=21
  PoI.Pos.z : Inport  Port=22
  PoI.Vel.x : Inport  Port=23
  PoI.Vel.y : Inport  Port=24
  PoI.Vel.z : Inport  Port=25
  PoI.Acc.x : Inport  Port=26
  PoI.Acc.y : Inport  Port=27
  PoI.Acc.z : Inport  Port=28
  PoI.Vel_1.x : Inport  Port=29
  PoI.Vel_1.y : Inport  Port=30
  PoI.Vel_1.z : Inport  Port=31
  PoI.Acc_1.x : Inport  Port=32
  PoI.Acc_1.y : Inport  Port=33
  PoI.Acc_1.z : Inport  Port=34
  PoI.GCS_Long : Inport  Port=35
  PoI.GCS_Lat : Inport  Port=36
  PoI.GCS_Elev : Inport  Port=37
  WheelOut.FL.t.x : Inport  Port=38
  WheelOut.FL.t.y : Inport  Port=39
  WheelOut.FL.t.z : Inport  Port=40
  WheelOut.FL.r_zxy.x : Inport  Port=41
  WheelOut.FL.r_zxy.y : Inport  Port=42
  WheelOut.FL.r_zxy.z : Inport  Port=43
  WheelOut.FL.Fx : Inport  Port=44
  WheelOut.FL.Fy : Inport  Port=45
  WheelOut.FL.Fz : Inport  Port=46
  WheelOut.FL.vBelt : Inport  Port=47
  WheelOut.FL.LongSlip : Inport  Port=48
  WheelOut.FL.SideSlip : Inport  Port=49
  WheelOut.FL.Trq_T2W : Inport  Port=50
  WheelOut.FL.Trq_WhlBearing : Inport  Port=51
  WheelOut.FR.t.x : Inport  Port=52
  WheelOut.FR.t.y : Inport  Port=53
  WheelOut.FR.t.z : Inport  Port=54
  WheelOut.FR.r_zxy.x : Inport  Port=55
  WheelOut.FR.r_zxy.y : Inport  Port=56
  WheelOut.FR.r_zxy.z : Inport  Port=57
  WheelOut.FR.Fx : Inport  Port=58
  WheelOut.FR.Fy : Inport  Port=59
  WheelOut.FR.Fz : Inport  Port=60
  WheelOut.FR.vBelt : Inport  Port=61
  WheelOut.FR.LongSlip : Inport  Port=62
  WheelOut.FR.SideSlip : Inport  Port=63
  WheelOut.FR.Trq_T2W : Inport  Port=64
  WheelOut.FR.Trq_WhlBearing : Inport  Port=65
  WheelOut.RL.t.x : Inport  Port=66
  WheelOut.RL.t.y : Inport  Port=67
  WheelOut.RL.t.z : Inport  Port=68
  WheelOut.RL.r_zxy.x : Inport  Port=69
  WheelOut.RL.r_zxy.y : Inport  Port=70
  WheelOut.RL.r_zxy.z : Inport  Port=71
  WheelOut.RL.Fx : Inport  Port=72
  WheelOut.RL.Fy : Inport  Port=73
  WheelOut.RL.Fz : Inport  Port=74
  WheelOut.RL.vBelt : Inport  Port=75
  WheelOut.RL.LongSlip : Inport  Port=76
  WheelOut.RL.SideSlip : Inport  Port=77
  WheelOut.RL.Trq_T2W : Inport  Port=78
  WheelOut.RL.Trq_WhlBearing : Inport  Port=79
  WheelOut.RR.t.x : Inport  Port=80
  WheelOut.RR.t.y : Inport  Port=81
  WheelOut.RR.t.z : Inport  Port=82
  WheelOut.RR.r_zxy.x : Inport  Port=83
  WheelOut.RR.r_zxy.y : Inport  Port=84
  WheelOut.RR.r_zxy.z : Inport  Port=85
  WheelOut.RR.Fx : Inport  Port=86
  WheelOut.RR.Fy : Inport  Port=87
  WheelOut.RR.Fz : Inport  Port=88
  WheelOut.RR.vBelt : Inport  Port=89
  WheelOut.RR.LongSlip : Inport  Port=90
  WheelOut.RR.SideSlip : Inport  Port=91
  WheelOut.RR.Trq_T2W : Inport  Port=92
  WheelOut.RR.Trq_WhlBearing : Inport  Port=93
  Fr1A.t_0.x : Inport  Port=94
  Fr1A.t_0.y : Inport  Port=95
  Fr1A.t_0.z : Inport  Port=96
  Fr1A.v_0.x : Inport  Port=97
  Fr1A.v_0.y : Inport  Port=98
  Fr1A.v_0.z : Inport  Port=99
  Fr1A.a_0.x : Inport  Port=100
  Fr1A.a_0.y : Inport  Port=101
  Fr1A.a_0.z : Inport  Port=102
  Fr1A.omega_0.x : Inport  Port=103
  Fr1A.omega_0.y : Inport  Port=104
  Fr1A.omega_0.z : Inport  Port=105
  Fr1A.alpha_0.x : Inport  Port=106
  Fr1A.alpha_0.y : Inport  Port=107
  Fr1A.alpha_0.z : Inport  Port=108
  Fr1A.Tr2Fr0.xx : Inport  Port=109
  Fr1A.Tr2Fr0.xy : Inport  Port=110
  Fr1A.Tr2Fr0.xz : Inport  Port=111
  Fr1A.Tr2Fr0.yx : Inport  Port=112
  Fr1A.Tr2Fr0.yy : Inport  Port=113
  Fr1A.Tr2Fr0.yz : Inport  Port=114
  Fr1A.Tr2Fr0.zx : Inport  Port=115
  Fr1A.Tr2Fr0.zy : Inport  Port=116
  Fr1A.Tr2Fr0.zz : Inport  Port=117
  AeroMarkerPos : BusCreator  Inputs=3
  AeroMarkerPos.x : Constant  Value=0
  AeroMarkerPos.y : Constant  Value=0
  AeroMarkerPos.z : Constant  Value=0
  Brake : BusCreator  Inputs=4
  Brake.FL : BusCreator  Inputs=3
  Brake.FL.Trq_BrakeReg_trg : Constant  Value=0
  Brake.FL.Trq_PB : Constant  Value=0
  Brake.FL.Trq_WB : Constant  Value=0
  Brake.FR : BusCreator  Inputs=3
  Brake.FR.Trq_BrakeReg_trg : Constant  Value=0
  Brake.FR.Trq_PB : Constant  Value=0
  Brake.FR.Trq_WB : Constant  Value=0
  Brake.RL : BusCreator  Inputs=3
  Brake.RL.Trq_BrakeReg_trg : Constant  Value=0
  Brake.RL.Trq_PB : Constant  Value=0
  Brake.RL.Trq_WB : Constant  Value=0
  Brake.RR : BusCreator  Inputs=3
  Brake.RR.Trq_BrakeReg_trg : Constant  Value=0
  Brake.RR.Trq_PB : Constant  Value=0
  Brake.RR.Trq_WB : Constant  Value=0
  Fr1A : BusCreator  Inputs=6
  Fr1A.Tr2Fr0 : BusCreator  Inputs=9
  Fr1A.a_0 : BusCreator  Inputs=3
  Fr1A.alpha_0 : BusCreator  Inputs=3
  Fr1A.omega_0 : BusCreator  Inputs=3
  Fr1A.t_0 : BusCreator  Inputs=3
  Fr1A.v_0 : BusCreator  Inputs=3
  Fr1B_r_xy : BusCreator  Inputs=2
  Fr1B_r_xy.x : Constant  Value=0
  Fr1B_r_xy.y : Constant  Value=0
  Hitch : BusCreator  Inputs=2
  Hitch.t_0 : BusCreator  Inputs=3
  Hitch.v_0 : BusCreator  Inputs=3
  Hitch.v_0.x : Constant  Value=0
  Hitch.v_0.y : Constant  Value=0
  Hitch.v_0.z : Constant  Value=0
  Motion : BusCreator  Inputs=13
  Motion.tRoad : Constant  Value=0
  PT : BusCreator  Inputs=10
  PT.DL_iDiff_mean : Constant  Value=0
  PT.Engine_rotv : Constant  Value=0
  PT.GearBox_GearNo : Constant  Value=0
  PT.Ignition : Constant  Value=0
  PT.OperationError : Constant  Value=0
  PT.OperationState : Constant  Value=0
  PT.Trq_Supp2Bdy1 : BusCreator  Inputs=3
  PT.Trq_Supp2Bdy1.x : Constant  Value=0
  PT.Trq_Supp2Bdy1.y : Constant  Value=0
  PT.Trq_Supp2Bdy1.z : Constant  Value=0
  PT.Trq_Supp2Bdy1B : BusCreator  Inputs=3
  PT.Trq_Supp2Bdy1B.x : Constant  Value=0
  PT.Trq_Supp2Bdy1B.y : Constant  Value=0
  PT.Trq_Supp2Bdy1B.z : Constant  Value=0
  PT.Trq_Supp2BdyEng : BusCreator  Inputs=2
  PT.Trq_Supp2BdyEng.x : Constant  Value=0
  PT.Trq_Supp2BdyEng.y : Constant  Value=0
  PT.Wheel : BusCreator  Inputs=4
  PT.Wheel.FL : BusCreator  Inputs=6
  PT.Wheel.FL.Trq_B2W : Constant  Value=0
  PT.Wheel.FL.Trq_BrakeReg : Constant  Value=0
  PT.Wheel.FL.Trq_BrakeReg_max : Constant  Value=0
  PT.Wheel.FL.Trq_Supp2WC : Constant  Value=0
  PT.Wheel.FL.rot : Constant  Value=0
  PT.Wheel.FL.rotv : Constant  Value=0
  PT.Wheel.FR : BusCreator  Inputs=6
  PT.Wheel.FR.Trq_B2W : Constant  Value=0
  PT.Wheel.FR.Trq_BrakeReg : Constant  Value=0
  PT.Wheel.FR.Trq_BrakeReg_max : Constant  Value=0
  PT.Wheel.FR.Trq_Supp2WC : Constant  Value=0
  PT.Wheel.FR.rot : Constant  Value=0
  PT.Wheel.FR.rotv : Constant  Value=0
  PT.Wheel.RL : BusCreator  Inputs=6
  PT.Wheel.RL.Trq_B2W : Constant  Value=0
  PT.Wheel.RL.Trq_BrakeReg : Constant  Value=0
  PT.Wheel.RL.Trq_BrakeReg_max : Constant  Value=0
  PT.Wheel.RL.Trq_Supp2WC : Constant  Value=0
  PT.Wheel.RL.rot : Constant  Value=0
  PT.Wheel.RL.rotv : Constant  Value=0
  PT.Wheel.RR : BusCreator  Inputs=6
  PT.Wheel.RR.Trq_B2W : Constant  Value=0
  PT.Wheel.RR.Trq_BrakeReg : Constant  Value=0
  PT.Wheel.RR.Trq_BrakeReg_max : Constant  Value=0
  PT.Wheel.RR.Trq_Supp2WC : Constant  Value=0
  PT.Wheel.RR.rot : Constant  Value=0
  PT.Wheel.RR.rotv : Constant  Value=0
  PoI : BusCreator  Inputs=8
  PoI.Acc : BusCreator  Inputs=3
  PoI.Acc_1 : BusCreator  Inputs=3
  PoI.Pos : BusCreator  Inputs=3
  PoI.Vel : BusCreator  Inputs=3
  PoI.Vel_1 : BusCreator  Inputs=3
  RateTransition : RateTransition  OutPortSampleTime=str2num(get_param(bdroot,'FixedStep'))
  Steering : BusCreator  Inputs=4
  WheelOut : BusCreator  Inputs=4
  WheelOut.FL : BusCreator  Inputs=15
  WheelOut.FL.FxTwin : Constant  Value=0
  WheelOut.FL.FyTwin : Constant  Value=0
  WheelOut.FL.FzTwin : Constant  Value=0
  WheelOut.FL.Trq_BrakeReg : Constant  Value=0
  WheelOut.FL.Trq_BrakeReg_max : Constant  Value=0
  WheelOut.FL.r_zxy : BusCreator  Inputs=3
  WheelOut.FL.t : BusCreator  Inputs=3
  WheelOut.FR : BusCreator  Inputs=15
  WheelOut.FR.FxTwin : Constant  Value=0
  WheelOut.FR.FyTwin : Constant  Value=0
  WheelOut.FR.FzTwin : Constant  Value=0
  WheelOut.FR.Trq_BrakeReg : Constant  Value=0
  WheelOut.FR.Trq_BrakeReg_max : Constant  Value=0
  WheelOut.FR.r_zxy : BusCreator  Inputs=3
  WheelOut.FR.t : BusCreator  Inputs=3
  WheelOut.RL : BusCreator  Inputs=15
  WheelOut.RL.FxTwin : Constant  Value=0
  WheelOut.RL.FyTwin : Constant  Value=0
  WheelOut.RL.FzTwin : Constant  Value=0
  WheelOut.RL.Trq_BrakeReg : Constant  Value=0
  WheelOut.RL.Trq_BrakeReg_max : Constant  Value=0
  WheelOut.RL.r_zxy : BusCreator  Inputs=3
  WheelOut.RL.t : BusCreator  Inputs=3
  WheelOut.RR : BusCreator  Inputs=15
  WheelOut.RR.FxTwin : Constant  Value=0
  WheelOut.RR.FyTwin : Constant  Value=0
  WheelOut.RR.FzTwin : Constant  Value=0
  WheelOut.RR.Trq_BrakeReg : Constant  Value=0
  WheelOut.RR.Trq_BrakeReg_max : Constant  Value=0
  WheelOut.RR.r_zxy : BusCreator  Inputs=3
  WheelOut.RR.t : BusCreator  Inputs=3
  cmVehicle_CarOut : BusCreator  Inputs=10
  ToCM : Outport  VectorParamsAs1DForOutWhenUnconnected=off
  wires:
  AeroMarkerPos.z/1 -> AeroMarkerPos/3  "z"
  AeroMarkerPos.y/1 -> AeroMarkerPos/2  "y"
  AeroMarkerPos.x/1 -> AeroMarkerPos/1  "x"
  AeroMarkerPos/1 -> cmVehicle_CarOut/10  "AeroMarkerPos"
  PT.Wheel.RR.Trq_BrakeReg_max/1 -> PT.Wheel.RR/6  "Trq_BrakeReg_max"
  PT.Wheel.RR.Trq_BrakeReg/1 -> PT.Wheel.RR/5  "Trq_BrakeReg"
  PT.Wheel.RR.Trq_Supp2WC/1 -> PT.Wheel.RR/4  "Trq_Supp2WC"
  PT.Wheel.RR.rotv/1 -> PT.Wheel.RR/3  "rotv"
  PT.Wheel.RR.rot/1 -> PT.Wheel.RR/2  "rot"
  PT.Wheel.RR.Trq_B2W/1 -> PT.Wheel.RR/1  "Trq_B2W"
  PT.Wheel.RR/1 -> PT.Wheel/4  "RR"
  PT.Wheel.RL.Trq_BrakeReg_max/1 -> PT.Wheel.RL/6  "Trq_BrakeReg_max"
  PT.Wheel.RL.Trq_BrakeReg/1 -> PT.Wheel.RL/5  "Trq_BrakeReg"
  PT.Wheel.RL.Trq_Supp2WC/1 -> PT.Wheel.RL/4  "Trq_Supp2WC"
  PT.Wheel.RL.rotv/1 -> PT.Wheel.RL/3  "rotv"
  PT.Wheel.RL.rot/1 -> PT.Wheel.RL/2  "rot"
  PT.Wheel.RL.Trq_B2W/1 -> PT.Wheel.RL/1  "Trq_B2W"
  PT.Wheel.RL/1 -> PT.Wheel/3  "RL"
  PT.Wheel.FR.Trq_BrakeReg_max/1 -> PT.Wheel.FR/6  "Trq_BrakeReg_max"
  PT.Wheel.FR.Trq_BrakeReg/1 -> PT.Wheel.FR/5  "Trq_BrakeReg"
  PT.Wheel.FR.Trq_Supp2WC/1 -> PT.Wheel.FR/4  "Trq_Supp2WC"
  PT.Wheel.FR.rotv/1 -> PT.Wheel.FR/3  "rotv"
  PT.Wheel.FR.rot/1 -> PT.Wheel.FR/2  "rot"
  PT.Wheel.FR.Trq_B2W/1 -> PT.Wheel.FR/1  "Trq_B2W"
  PT.Wheel.FR/1 -> PT.Wheel/2  "FR"
  PT.Wheel.FL.Trq_BrakeReg_max/1 -> PT.Wheel.FL/6  "Trq_BrakeReg_max"
  PT.Wheel.FL.Trq_BrakeReg/1 -> PT.Wheel.FL/5  "Trq_BrakeReg"
  PT.Wheel.FL.Trq_Supp2WC/1 -> PT.Wheel.FL/4  "Trq_Supp2WC"
  PT.Wheel.FL.rotv/1 -> PT.Wheel.FL/3  "rotv"
  PT.Wheel.FL.rot/1 -> PT.Wheel.FL/2  "rot"
  PT.Wheel.FL.Trq_B2W/1 -> PT.Wheel.FL/1  "Trq_B2W"
  PT.Wheel.FL/1 -> PT.Wheel/1  "FL"
  PT.Wheel/1 -> PT/10  "Wheel"
  PT.DL_iDiff_mean/1 -> PT/9  "DL_iDiff_mean"
  PT.GearBox_GearNo/1 -> PT/8  "GearBox_GearNo"
  PT.Engine_rotv/1 -> PT/7  "Engine_rotv"
  PT.OperationError/1 -> PT/6  "OperationError"
  PT.OperationState/1 -> PT/5  "OperationState"
  PT.Ignition/1 -> PT/4  "Ignition"
  PT.Trq_Supp2BdyEng.y/1 -> PT.Trq_Supp2BdyEng/2  "y"
  PT.Trq_Supp2BdyEng.x/1 -> PT.Trq_Supp2BdyEng/1  "x"
  PT.Trq_Supp2BdyEng/1 -> PT/3  "Trq_Supp2BdyEng"
  PT.Trq_Supp2Bdy1B.z/1 -> PT.Trq_Supp2Bdy1B/3  "z"
  PT.Trq_Supp2Bdy1B.y/1 -> PT.Trq_Supp2Bdy1B/2  "y"
  PT.Trq_Supp2Bdy1B.x/1 -> PT.Trq_Supp2Bdy1B/1  "x"
  PT.Trq_Supp2Bdy1B/1 -> PT/2  "Trq_Supp2Bdy1B"
  PT.Trq_Supp2Bdy1.z/1 -> PT.Trq_Supp2Bdy1/3  "z"
  PT.Trq_Supp2Bdy1.y/1 -> PT.Trq_Supp2Bdy1/2  "y"
  PT.Trq_Supp2Bdy1.x/1 -> PT.Trq_Supp2Bdy1/1  "x"
  PT.Trq_Supp2Bdy1/1 -> PT/1  "Trq_Supp2Bdy1"
  PT/1 -> cmVehicle_CarOut/9  "PT"
  Brake.RR.Trq_BrakeReg_trg/1 -> Brake.RR/3  "Trq_BrakeReg_trg"
  Brake.RR.Trq_PB/1 -> Brake.RR/2  "Trq_PB"
  Brake.RR.Trq_WB/1 -> Brake.RR/1  "Trq_WB"
  Brake.RR/1 -> Brake/4  "RR"
  Brake.RL.Trq_BrakeReg_trg/1 -> Brake.RL/3  "Trq_BrakeReg_trg"
  Brake.RL.Trq_PB/1 -> Brake.RL/2  "Trq_PB"
  Brake.RL.Trq_WB/1 -> Brake.RL/1  "Trq_WB"
  Brake.RL/1 -> Brake/3  "RL"
  Brake.FR.Trq_BrakeReg_trg/1 -> Brake.FR/3  "Trq_BrakeReg_trg"
  Brake.FR.Trq_PB/1 -> Brake.FR/2  "Trq_PB"
  Brake.FR.Trq_WB/1 -> Brake.FR/1  "Trq_WB"
  Brake.FR/1 -> Brake/2  "FR"
  Brake.FL.Trq_BrakeReg_trg/1 -> Brake.FL/3  "Trq_BrakeReg_trg"
  Brake.FL.Trq_PB/1 -> Brake.FL/2  "Trq_PB"
  Brake.FL.Trq_WB/1 -> Brake.FL/1  "Trq_WB"
  Brake.FL/1 -> Brake/1  "FL"
  Brake/1 -> cmVehicle_CarOut/8  "Brake"
  Fr1B_r_xy.y/1 -> Fr1B_r_xy/2  "y"
  Fr1B_r_xy.x/1 -> Fr1B_r_xy/1  "x"
  Fr1B_r_xy/1 -> cmVehicle_CarOut/7  "Fr1B_r_xy"
  Fr1A.Tr2Fr0/1 -> Fr1A/6  "Tr2Fr0"
  Fr1A.alpha_0/1 -> Fr1A/5  "alpha_0"
  Fr1A.omega_0/1 -> Fr1A/4  "omega_0"
  Fr1A.a_0/1 -> Fr1A/3  "a_0"
  Fr1A.v_0/1 -> Fr1A/2  "v_0"
  Fr1A.t_0/1 -> Fr1A/1  "t_0"
  Fr1A/1 -> cmVehicle_CarOut/6  "Fr1A"
  WheelOut.RR.Trq_BrakeReg_max/1 -> WheelOut.RR/15  "Trq_BrakeReg_max"
  WheelOut.RR.Trq_BrakeReg/1 -> WheelOut.RR/14  "Trq_BrakeReg"
  WheelOut.RR.FzTwin/1 -> WheelOut.RR/10  "FzTwin"
  WheelOut.RR.FyTwin/1 -> WheelOut.RR/9  "FyTwin"
  WheelOut.RR.FxTwin/1 -> WheelOut.RR/8  "FxTwin"
  WheelOut.RR.r_zxy/1 -> WheelOut.RR/2  "r_zxy"
  WheelOut.RR.t/1 -> WheelOut.RR/1  "t"
  WheelOut.RR/1 -> WheelOut/4  "RR"
  WheelOut.RL.Trq_BrakeReg_max/1 -> WheelOut.RL/15  "Trq_BrakeReg_max"
  WheelOut.RL.Trq_BrakeReg/1 -> WheelOut.RL/14  "Trq_BrakeReg"
  WheelOut.RL.FzTwin/1 -> WheelOut.RL/10  "FzTwin"
  WheelOut.RL.FyTwin/1 -> WheelOut.RL/9  "FyTwin"
  WheelOut.RL.FxTwin/1 -> WheelOut.RL/8  "FxTwin"
  WheelOut.RL.r_zxy/1 -> WheelOut.RL/2  "r_zxy"
  WheelOut.RL.t/1 -> WheelOut.RL/1  "t"
  WheelOut.RL/1 -> WheelOut/3  "RL"
  WheelOut.FR.Trq_BrakeReg_max/1 -> WheelOut.FR/15  "Trq_BrakeReg_max"
  WheelOut.FR.Trq_BrakeReg/1 -> WheelOut.FR/14  "Trq_BrakeReg"
  WheelOut.FR.FzTwin/1 -> WheelOut.FR/10  "FzTwin"
  WheelOut.FR.FyTwin/1 -> WheelOut.FR/9  "FyTwin"
  WheelOut.FR.FxTwin/1 -> WheelOut.FR/8  "FxTwin"
  WheelOut.FR.r_zxy/1 -> WheelOut.FR/2  "r_zxy"
  WheelOut.FR.t/1 -> WheelOut.FR/1  "t"
  WheelOut.FR/1 -> WheelOut/2  "FR"
  WheelOut.FL.Trq_BrakeReg_max/1 -> WheelOut.FL/15  "Trq_BrakeReg_max"
  WheelOut.FL.Trq_BrakeReg/1 -> WheelOut.FL/14  "Trq_BrakeReg"
  WheelOut.FL.FzTwin/1 -> WheelOut.FL/10  "FzTwin"
  WheelOut.FL.FyTwin/1 -> WheelOut.FL/9  "FyTwin"
  WheelOut.FL.FxTwin/1 -> WheelOut.FL/8  "FxTwin"
  WheelOut.FL.r_zxy/1 -> WheelOut.FL/2  "r_zxy"
  WheelOut.FL.t/1 -> WheelOut.FL/1  "t"
  WheelOut.FL/1 -> WheelOut/1  "FL"
  WheelOut/1 -> cmVehicle_CarOut/5  "WheelOut"
  PoI.Acc_1/1 -> PoI/8  "Acc_1"
  PoI.Vel_1/1 -> PoI/7  "Vel_1"
  PoI.Acc/1 -> PoI/3  "Acc"
  PoI.Vel/1 -> PoI/2  "Vel"
  PoI.Pos/1 -> PoI/1  "Pos"
  PoI/1 -> cmVehicle_CarOut/4  "PoI"
  Hitch.v_0.z/1 -> Hitch.v_0/3  "z"
  Hitch.v_0.y/1 -> Hitch.v_0/2  "y"
  Hitch.v_0.x/1 -> Hitch.v_0/1  "x"
  Hitch.v_0/1 -> Hitch/2  "v_0"
  Hitch.t_0/1 -> Hitch/1  "t_0"
  Hitch/1 -> cmVehicle_CarOut/3  "Hitch"
  Motion.tRoad/1 -> Motion/2  "tRoad"
  Motion/1 -> cmVehicle_CarOut/2  "Motion"
  Steering/1 -> cmVehicle_CarOut/1  "Steering"
  cmVehicle_CarOut/1 -> RateTransition/1
  RateTransition/1 -> ToCM/1
  Steering.Ang/1 -> Steering/1  "Ang"
  Steering.AngVel/1 -> Steering/2  "AngVel"
  Steering.AngAcc/1 -> Steering/3  "AngAcc"
  Steering.Trq/1 -> Steering/4  "Trq"
  Motion.v/1 -> Motion/4  "v"
  Motion.Distance/1 -> Motion/3  "Distance"
  Motion.sRoad/1 -> Motion/1  "sRoad"
  Motion.Roll/1 -> Motion/8  "Roll"
  Motion.RollVel/1 -> Motion/9  "RollVel"
  Motion.RollAcc/1 -> Motion/10  "RollAcc"
  Motion.Pitch/1 -> Motion/11  "Pitch"
  Motion.PitchVel/1 -> Motion/12  "PitchVel"
  Motion.PitchAcc/1 -> Motion/13  "PitchAcc"
  Motion.Yaw/1 -> Motion/5  "Yaw"
  Motion.YawRate/1 -> Motion/6  "YawRate"
  Motion.YawAcc/1 -> Motion/7  "YawAcc"
  Hitch.t_0.x/1 -> Hitch.t_0/1  "x"
  Hitch.t_0.y/1 -> Hitch.t_0/2  "y"
  Hitch.t_0.z/1 -> Hitch.t_0/3  "z"
  PoI.Pos.x/1 -> PoI.Pos/1  "x"
  PoI.Pos.y/1 -> PoI.Pos/2  "y"
  PoI.Pos.z/1 -> PoI.Pos/3  "z"
  PoI.Vel.x/1 -> PoI.Vel/1  "x"
  PoI.Vel.y/1 -> PoI.Vel/2  "y"
  PoI.Vel.z/1 -> PoI.Vel/3  "z"
  PoI.Acc.x/1 -> PoI.Acc/1  "x"
  PoI.Acc.y/1 -> PoI.Acc/2  "y"
  PoI.Acc.z/1 -> PoI.Acc/3  "z"
  PoI.Vel_1.x/1 -> PoI.Vel_1/1  "x"
  PoI.Vel_1.y/1 -> PoI.Vel_1/2  "y"
  PoI.Vel_1.z/1 -> PoI.Vel_1/3  "z"
  PoI.Acc_1.x/1 -> PoI.Acc_1/1  "x"
  PoI.Acc_1.y/1 -> PoI.Acc_1/2  "y"
  PoI.Acc_1.z/1 -> PoI.Acc_1/3  "z"
  PoI.GCS_Long/1 -> PoI/4  "GCS_Long"
  PoI.GCS_Lat/1 -> PoI/5  "GCS_Lat"
  PoI.GCS_Elev/1 -> PoI/6  "GCS_Elev"
  WheelOut.FL.t.x/1 -> WheelOut.FL.t/1  "x"
  WheelOut.FL.t.y/1 -> WheelOut.FL.t/2  "y"
  WheelOut.FL.t.z/1 -> WheelOut.FL.t/3  "z"
  WheelOut.FL.r_zxy.x/1 -> WheelOut.FL.r_zxy/1  "x"
  WheelOut.FL.r_zxy.y/1 -> WheelOut.FL.r_zxy/2  "y"
  WheelOut.FL.r_zxy.z/1 -> WheelOut.FL.r_zxy/3  "z"
  WheelOut.FL.Fx/1 -> WheelOut.FL/5  "Fx"
  WheelOut.FL.Fy/1 -> WheelOut.FL/6  "Fy"
  WheelOut.FL.Fz/1 -> WheelOut.FL/7  "Fz"
  WheelOut.FL.vBelt/1 -> WheelOut.FL/13  "vBelt"
  WheelOut.FL.LongSlip/1 -> WheelOut.FL/3  "LongSlip"
  WheelOut.FL.SideSlip/1 -> WheelOut.FL/4  "SideSlip"
  WheelOut.FL.Trq_T2W/1 -> WheelOut.FL/11  "Trq_T2W"
  WheelOut.FL.Trq_WhlBearing/1 -> WheelOut.FL/12  "Trq_WhlBearing"
  WheelOut.FR.t.x/1 -> WheelOut.FR.t/1  "x"
  WheelOut.FR.t.y/1 -> WheelOut.FR.t/2  "y"
  WheelOut.FR.t.z/1 -> WheelOut.FR.t/3  "z"
  WheelOut.FR.r_zxy.x/1 -> WheelOut.FR.r_zxy/1  "x"
  WheelOut.FR.r_zxy.y/1 -> WheelOut.FR.r_zxy/2  "y"
  WheelOut.FR.r_zxy.z/1 -> WheelOut.FR.r_zxy/3  "z"
  WheelOut.FR.Fx/1 -> WheelOut.FR/5  "Fx"
  WheelOut.FR.Fy/1 -> WheelOut.FR/6  "Fy"
  WheelOut.FR.Fz/1 -> WheelOut.FR/7  "Fz"
  WheelOut.FR.vBelt/1 -> WheelOut.FR/13  "vBelt"
  WheelOut.FR.LongSlip/1 -> WheelOut.FR/3  "LongSlip"
  WheelOut.FR.SideSlip/1 -> WheelOut.FR/4  "SideSlip"
  WheelOut.FR.Trq_T2W/1 -> WheelOut.FR/11  "Trq_T2W"
  WheelOut.FR.Trq_WhlBearing/1 -> WheelOut.FR/12  "Trq_WhlBearing"
  WheelOut.RL.t.x/1 -> WheelOut.RL.t/1  "x"
  WheelOut.RL.t.y/1 -> WheelOut.RL.t/2  "y"
  WheelOut.RL.t.z/1 -> WheelOut.RL.t/3  "z"
  WheelOut.RL.r_zxy.x/1 -> WheelOut.RL.r_zxy/1  "x"
  WheelOut.RL.r_zxy.y/1 -> WheelOut.RL.r_zxy/2  "y"
  WheelOut.RL.r_zxy.z/1 -> WheelOut.RL.r_zxy/3  "z"
  WheelOut.RL.Fx/1 -> WheelOut.RL/5  "Fx"
  WheelOut.RL.Fy/1 -> WheelOut.RL/6  "Fy"
  WheelOut.RL.Fz/1 -> WheelOut.RL/7  "Fz"
  WheelOut.RL.LongSlip/1 -> WheelOut.RL/3  "LongSlip"
  WheelOut.RL.SideSlip/1 -> WheelOut.RL/4  "SideSlip"
  WheelOut.RL.Trq_T2W/1 -> WheelOut.RL/11  "Trq_T2W"
  WheelOut.RL.Trq_WhlBearing/1 -> WheelOut.RL/12  "Trq_WhlBearing"
  WheelOut.RR.t.x/1 -> WheelOut.RR.t/1  "x"
  WheelOut.RR.t.y/1 -> WheelOut.RR.t/2  "y"
  WheelOut.RR.t.z/1 -> WheelOut.RR.t/3  "z"
  WheelOut.RR.r_zxy.x/1 -> WheelOut.RR.r_zxy/1  "x"
  WheelOut.RR.r_zxy.y/1 -> WheelOut.RR.r_zxy/2  "y"
  WheelOut.RR.r_zxy.z/1 -> WheelOut.RR.r_zxy/3  "z"
  WheelOut.RR.Fx/1 -> WheelOut.RR/5  "Fx"
  WheelOut.RR.Fy/1 -> WheelOut.RR/6  "Fy"
  WheelOut.RR.Fz/1 -> WheelOut.RR/7  "Fz"
  WheelOut.RR.LongSlip/1 -> WheelOut.RR/3  "LongSlip"
  WheelOut.RR.SideSlip/1 -> WheelOut.RR/4  "SideSlip"
  WheelOut.RR.Trq_T2W/1 -> WheelOut.RR/11  "Trq_T2W"
  WheelOut.RR.Trq_WhlBearing/1 -> WheelOut.RR/12  "Trq_WhlBearing"
  WheelOut.RL.vBelt/1 -> WheelOut.RL/13  "vBelt"
  WheelOut.RR.vBelt/1 -> WheelOut.RR/13  "vBelt"
  Fr1A.t_0.x/1 -> Fr1A.t_0/1  "x"
  Fr1A.t_0.y/1 -> Fr1A.t_0/2  "y"
  Fr1A.t_0.z/1 -> Fr1A.t_0/3  "z"
  Fr1A.v_0.x/1 -> Fr1A.v_0/1  "x"
  Fr1A.v_0.y/1 -> Fr1A.v_0/2  "y"
  Fr1A.v_0.z/1 -> Fr1A.v_0/3  "z"
  Fr1A.a_0.x/1 -> Fr1A.a_0/1  "x"
  Fr1A.a_0.y/1 -> Fr1A.a_0/2  "y"
  Fr1A.a_0.z/1 -> Fr1A.a_0/3  "z"
  Fr1A.omega_0.x/1 -> Fr1A.omega_0/1  "x"
  Fr1A.omega_0.y/1 -> Fr1A.omega_0/2  "y"
  Fr1A.omega_0.z/1 -> Fr1A.omega_0/3  "z"
  Fr1A.alpha_0.x/1 -> Fr1A.alpha_0/1  "x"
  Fr1A.alpha_0.y/1 -> Fr1A.alpha_0/2  "y"
  Fr1A.alpha_0.z/1 -> Fr1A.alpha_0/3  "z"
  Fr1A.Tr2Fr0.xx/1 -> Fr1A.Tr2Fr0/1  "xx"
  Fr1A.Tr2Fr0.xy/1 -> Fr1A.Tr2Fr0/2  "xy"
  Fr1A.Tr2Fr0.xz/1 -> Fr1A.Tr2Fr0/3  "xz"
  Fr1A.Tr2Fr0.yx/1 -> Fr1A.Tr2Fr0/4  "yx"
  Fr1A.Tr2Fr0.yy/1 -> Fr1A.Tr2Fr0/5  "yy"
  Fr1A.Tr2Fr0.yz/1 -> Fr1A.Tr2Fr0/6  "yz"
  Fr1A.Tr2Fr0.zx/1 -> Fr1A.Tr2Fr0/7  "zx"
  Fr1A.Tr2Fr0.zy/1 -> Fr1A.Tr2Fr0/8  "zy"
  Fr1A.Tr2Fr0.zz/1 -> Fr1A.Tr2Fr0/9  "zz"

== system UserVehicle_RTW/SingleTrack_Out/Subsystem ==
  In1 : Inport
  Bus Creator{,1..4} (5 alike) : BusCreator  Inputs=3
  foo_Input_Selector2 : BusSelector  OutputSignals=Vhcl PoI_Pos x,Vhcl PoI_Pos y,Vhcl PoI_Pos z,Vhcl PoI_Vel x,Vhcl PoI_Vel y,Vhcl PoI_Vel z,Vhcl PoI_Acc x,Vhcl PoI_Acc y,Vhcl PoI_Acc z,Vhcl PoI_Vel_1 x,Vhcl PoI_Vel_1 y,Vhcl PoI_Vel_1 z,Vhcl PoI_Acc_1 x,Vhcl PoI_Acc_1 y,Vhcl PoI_Acc_1 z,Vhcl PoI_GCS Long,Vhcl PoI_GCS Lat,Vhcl PoI_GCS Elev
  Out1 : Outport  VectorParamsAs1DForOutWhenUnconnected=off
  Out2 : Outport  Port=2  VectorParamsAs1DForOutWhenUnconnected=off
  Out3 : Outport  Port=3  VectorParamsAs1DForOutWhenUnconnected=off
  Out4 : Outport  Port=4  VectorParamsAs1DForOutWhenUnconnected=off
  Out5 : Outport  Port=5  VectorParamsAs1DForOutWhenUnconnected=off
  Out6 : Outport  Port=6  VectorParamsAs1DForOutWhenUnconnected=off
  Out7 : Outport  Port=7  VectorParamsAs1DForOutWhenUnconnected=off
  Out8 : Outport  Port=8  VectorParamsAs1DForOutWhenUnconnected=off
  wires:
  foo_Input_Selector2/1 -> Bus Creator/1  "<Vhcl PoI_Pos x>"
  foo_Input_Selector2/2 -> Bus Creator/2  "<Vhcl PoI_Pos y>"
  foo_Input_Selector2/3 -> Bus Creator/3  "<Vhcl PoI_Pos z>"
  foo_Input_Selector2/4 -> Bus Creator1/1  "<Vhcl PoI_Vel x>"
  foo_Input_Selector2/5 -> Bus Creator1/2  "<Vhcl PoI_Vel y>"
  foo_Input_Selector2/6 -> Bus Creator1/3  "<Vhcl PoI_Vel z>"
  foo_Input_Selector2/7 -> Bus Creator2/1  "<Vhcl PoI_Acc x>"
  foo_Input_Selector2/8 -> Bus Creator2/2  "<Vhcl PoI_Acc y>"
  foo_Input_Selector2/9 -> Bus Creator2/3  "<Vhcl PoI_Acc z>"
  foo_Input_Selector2/10 -> Bus Creator3/1  "<Vhcl PoI_Vel_1 x>"
  foo_Input_Selector2/11 -> Bus Creator3/2  "<Vhcl PoI_Vel_1 y>"
  foo_Input_Selector2/12 -> Bus Creator3/3  "<Vhcl PoI_Vel_1 z>"
  foo_Input_Selector2/13 -> Bus Creator4/1  "<Vhcl PoI_Acc_1 x>"
  foo_Input_Selector2/14 -> Bus Creator4/2  "<Vhcl PoI_Acc_1 y>"
  foo_Input_Selector2/15 -> Bus Creator4/3  "<Vhcl PoI_Acc_1 z>"
  Bus Creator/1 -> Out1/1
  Bus Creator1/1 -> Out2/1
  Bus Creator2/1 -> Out3/1
  In1/1 -> foo_Input_Selector2/1
  Bus Creator3/1 -> Out4/1
  Bus Creator4/1 -> Out5/1
  foo_Input_Selector2/16 -> Out6/1  "<Vhcl PoI_GCS Long>"
  foo_Input_Selector2/17 -> Out7/1  "<Vhcl PoI_GCS Lat>"
  foo_Input_Selector2/18 -> Out8/1  "<Vhcl PoI_GCS Elev>"
